simulink model "ExperimentModelPIDDigital"  (R2020b)
settings: Solver=FixedStepDiscrete  StartTime=0.0  StopTime=10  FixedStep=Ts  RelTol=1e-3
undefined symbols (not defined in the file): CDer, CInt, finalValue, Kd, Ki, Kp, National_Instruments, PCI, sens, Ts
libraries: sldrtlib x3
settings Model: ExtModeTrigDuration=100000  Creator=umbe  LastModifiedBy=Diego
settings DataIOCC: ReturnWorkspaceOutputs=off
settings RTWCC: Description=Simulink Desktop Real-Time  SystemTargetFile=sldrt.tlc  TemplateMakefile=sldrt.tmf  RTWCompilerOptimization=on
settings CodeAppCC: MaxIdLength=95
settings SimulinkDesktopRealTimeCC: TargetPreCompLibLocation=C:\Program Files\MATLAB\R2020b\toolbox\sldrt\lib\win64

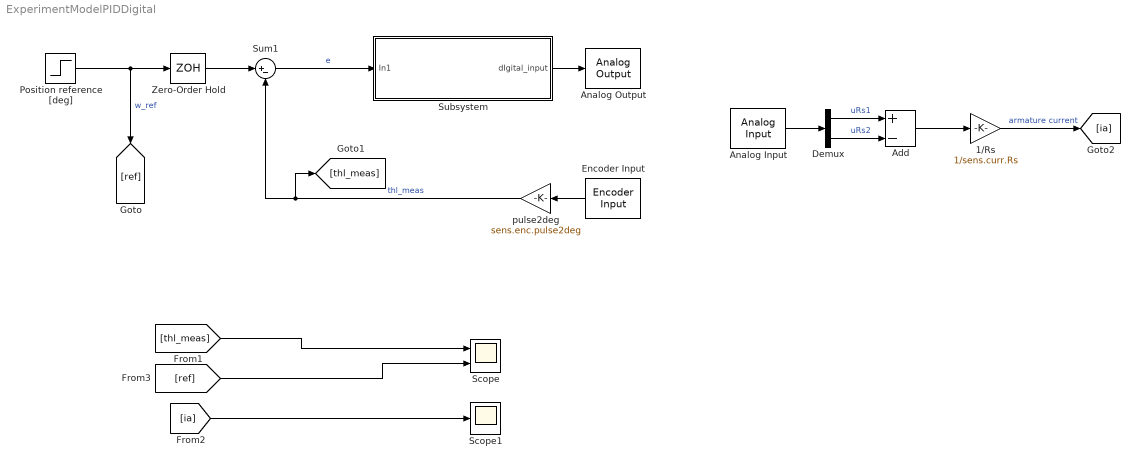
== system ExperimentModelPIDDigital ==
  1/Rs : Gain  Gain=1/sens.curr.Rs
  Add : Sum  Inputs=+-
  Analog Input : sldrtlib/Analog Input  SampleTime=Ts  MaxMissedTicks=10  ShowMissedTicks=off  YieldWhenWaiting=off  DrvName=National_Instruments/PCI-6221  DrvAddress=4294967295  DrvOptions=[0 0 0 2 0]  Channels=[1 2]  RangeMode=1  VoltRange=1  DataType=1
      settings: AttributesFormatString=National Instruments\nPCI-6221 [auto]
  Analog Output : sldrtlib/Analog Output  SampleTime=Ts  MaxMissedTicks=10  ShowMissedTicks=off  YieldWhenWaiting=off  DrvName=National_Instruments/PCI-6221  DrvAddress=4294967295  DrvOptions=[0 0 0 2 0]  Channels=1  RangeMode=1  VoltRange=1  InitialValue=0  FinalValue=0
      settings: AttributesFormatString=National Instruments\nPCI-6221 [auto]
  Demux : Demux  Outputs=2
  Encoder Input : sldrtlib/Encoder Input  SampleTime=Ts  MaxMissedTicks=10  ShowMissedTicks=off  YieldWhenWaiting=off  DrvName=National_Instruments/PCI-6221  DrvAddress=4294967295  DrvOptions=[0 0 0 2 0]  Channels=1  QuadMode=3  IndexPulse=1  InputFilter=Inf  DataType=1
      settings: AttributesFormatString=National Instruments\nPCI-6221 [auto]
  Position reference [deg] : Step  After=finalValue  SampleTime=0
  Scope : Scope  NumInputPorts=2
  Scope1 : Scope
  Subsystem : Subsystem
  Sum1 : Sum  Inputs=|+-
  Zero-Order Hold : ZeroOrderHold  SampleTime=Ts
  pulse2deg : Gain  Gain=sens.enc.pulse2deg
  wires:
  1/Rs/1 -> [ia]  "armature current"
  Add/1 -> 1/Rs/1
  Demux/1 -> Add/1  "uRs1"
  Demux/2 -> Add/2  "uRs2"
  pulse2deg/1 -> [thl_meas], Sum1/2  "thl_meas"
  Sum1/1 -> Subsystem/1(In1)  "e"
  [thl_meas] -> Scope/1
  [ia] -> Scope1/1
  Encoder Input/1 -> pulse2deg/1
  Analog Input/1 -> Demux/1
  Subsystem/1(dIgital_input) -> Analog Output/1
  Position reference [deg]/1 -> Zero-Order Hold/1, [ref]  "w_ref"
  Zero-Order Hold/1 -> Sum1/1
  [ref] -> Scope/2

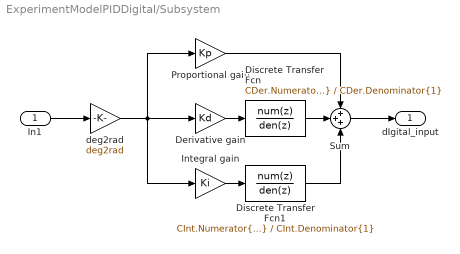
== system ExperimentModelPIDDigital/Subsystem ==
  In1 : Inport
  Derivative gain : Gain  Gain=Kd
  Discrete Transfer Fcn : DiscreteTransferFcn  Numerator=CDer.Numerator{1}  Denominator=CDer.Denominator{1}  SampleTime=Ts
  Discrete Transfer Fcn1 : DiscreteTransferFcn  Numerator=CInt.Numerator{1}  Denominator=CInt.Denominator{1}  SampleTime=Ts
  Integral gain : Gain  Gain=Ki
  Proportional gain : Gain  Gain=Kp
  Sum : Sum  Inputs=+++
  deg2rad : Gain  Gain=deg2rad
  dIgital_input : Outport
  wires:
  Integral gain/1 -> Discrete Transfer Fcn1/1
  Discrete Transfer Fcn1/1 -> Sum/3
  Proportional gain/1 -> Sum/1
  Discrete Transfer Fcn/1 -> Sum/2
  Derivative gain/1 -> Discrete Transfer Fcn/1
  Sum/1 -> dIgital_input/1
  deg2rad/1 -> Integral gain/1, Derivative gain/1, Proportional gain/1
  In1/1 -> deg2rad/1
